simulink model "ModelD"  (R2014a)
settings: Solver=FixedStepDiscrete  StartTime=0.0  StopTime=10.0  RelTol=1e-3
libraries: simulink x8
settings Model: SimulationMode=external  ExtModeTrigDuration=100  Creator=admin  LastModifiedBy=admin
settings SolverCC: AutoInsertRateTranBlk=on
settings DataIOCC: SaveOutput=off  SaveTime=off
settings OptimizationCC: InlineParams=on  InlineInvariantSignals=on  StateBitsets=on  DataBitsets=on  UseTempVars=on  ZeroExternalMemoryAtStartup=off  ZeroInternalMemoryAtStartup=off  NoFixptDivByZeroProtection=on  EfficientFloat2IntCast=on  OptimizeModelRefInitCode=on  LifeSpan=1
settings DebuggingCC: SolverPrmCheckMsg=none
settings HardwareCC: ProdLargestAtomicInteger=Long  ProdLargestAtomicFloat=Double  ProdEndianess=LittleEndian  ProdHWDeviceType=ARM Compatible->ARM Cortex
settings RTWCC: SystemTargetFile=realtime.tlc  TLCOptions=-p0  GenCodeOnly=on  GenerateMakefile=off  TemplateMakefile=realtime.tmf  Description=Run on Target Hardware  RTWVerbose=off  ProcessScript=realtime_make_rtw_hook  IncludeHyperlinkInReport=on
settings CodeAppCC: ForceParamTrailComments=on  SimulinkDataObjDesc=on  CustomSymbolStrGlobalVar=rt$N$M  CustomSymbolStrType=$N$M  CustomSymbolStrFcn=$N$M$F  CustomSymbolStrMacro=$N$M  InsertBlockDesc=on
settings STFCustomTargetCC: TargetLibSuffix=.a  GenerateSampleERTMain=on  ConcurrentExecutionCompliant=off  GeneratePreprocessorConditionals=Use local settings  ERTCustomFileBanners=on  SupportNonInlinedSFcns=off  SupportVariableSizeSignals=on  MATLABClassNameForMDSCustomization=Simulink.SoftwareTarget.ERTCustomization  GRTInterface=off  SystemTargetFile=realtime.tlc
settings ERTTargetCC: CombineOutputUpdateFcns=off  SupportContinuousTime=on  SupportVariableSizeSignals=on  ExtModeMexArgs='localhost' 0 17725  ERTSrcFileBannerTemplate=realtime_code_template.cgt  ERTHdrFileBannerTemplate=realtime_code_template.cgt  ERTDataSrcFileTemplate=realtime_code_template.cgt  ERTDataHdrFileTemplate=realtime_code_template.cgt  ERTCustomFileTemplate=realtime_file_process.tlc

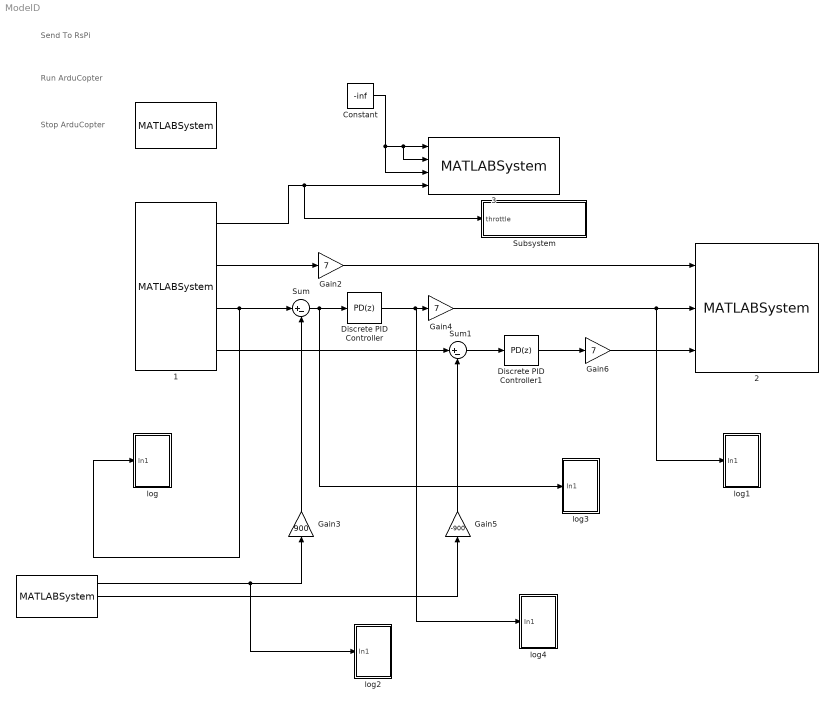
== system ModelD ==
  note: Send To RsPi
  note: Run ArduCopter
  note: Stop ArduCopter
  "  " : MATLABSystem  System=Gyro  SimulateUsing=Interpreted execution
      mask Type: Gyro
      mask Display:
      | disp('Gyro');
      | port_label('output',1,'x');
      | port_label('output',2,'y');
      | port_label('output',3,'z');
  "   " : MATLABSystem  System=Accel  SimulateUsing=Interpreted execution
      mask Type: Accel
      mask Display:
      | disp('Accel');
      | port_label('output',1,'x');
      | port_label('output',2,'y');
      | port_label('output',3,'z');
  "   1" : MATLABSystem  System=RC  SimulateUsing=Interpreted execution
      mask Type: RC
      mask Display:
      | disp('RC');
      | port_label('output',1,'thort');
      | port_label('output',2,'yawR');
      | port_label('output',3,'pitch');
      | port_label('output',4,'roll');
  "   2" : MATLABSystem  System=RateController  SimulateUsing=Interpreted execution
      mask Type: RateController
      mask Display:
      | disp('RateController');
      | port_label('input',1,'yaw');
      | port_label('input',2,'pitch');
      | port_label('input',3,'roll');
  "   3" : MATLABSystem  System=Motors  SimulateUsing=Interpreted execution
      mask Type: Motors
      mask Display:
      | disp('Motors');
      | port_label('input',1,'roll');
      | port_label('input',2,'pitch');
      | port_label('input',3,'yaw');
      | port_label('input',4,'throttle');
  Constant : Constant  Value=-inf
  Discrete PID Controller : simulink/Continuous/PID Controller  Controller=PD  TimeDomain=Discrete-time  SampleTime=-1  IntegratorMethod=Forward Euler  FilterMethod=Forward Euler  Form=Parallel  P=1  I=0  D=0.1  N=3  InitialConditionSource=internal  InitialConditionForIntegrator=0  InitialConditionForFilter=0  ExternalReset=none  ZeroCross=off  LimitOutput=off  UpperSaturationLimit=inf  LowerSaturationLimit=-inf  LinearizeAsGain=off  AntiWindupMode=none  Kb=1  TrackingMode=off  Kt=1  PParamMin=[]  PParamMax=[]  IParamMin=[]  IParamMax=[]  DParamMin=[]  DParamMax=[]  NParamMin=[]  NParamMax=[]  KbParamMin=[]  KbParamMax=[]  KtParamMin=[]  KtParamMax=[]  POutMin=[]  POutMax=[]  IOutMin=[]  IOutMax=[]  DOutMin=[]  DOutMax=[]  NOutMin=[]  NOutMax=[]  KbOutMin=[]  KbOutMax=[]  KtOutMin=[]  KtOutMax=[]  IntegratorOutMin=[]  IntegratorOutMax=[]  FilterOutMin=[]  FilterOutMax=[]  SumOutMin=[]  SumOutMax=[]  SumI1OutMin=[]  SumI1OutMax=[]  SumI2OutMin=[]  SumI2OutMax=[]  SumI3OutMin=[]  SumI3OutMax=[]  SumDOutMin=[]  SumDOutMax=[]  SaturationOutMin=[]  SaturationOutMax=[]  IntegratorContinuousStateAttributes=''  IntegratorStateMustResolveToSignalObject=off  IntegratorRTWStateStorageClass=Auto  FilterContinuousStateAttributes=''  FilterStateMustResolveToSignalObject=off  FilterRTWStateStorageClass=Auto
  Discrete PID Controller1 : simulink/Continuous/PID Controller  Controller=PD  TimeDomain=Discrete-time  SampleTime=-1  IntegratorMethod=Forward Euler  FilterMethod=Forward Euler  Form=Parallel  P=1  I=0  D=0.1  N=3  InitialConditionSource=internal  InitialConditionForIntegrator=0  InitialConditionForFilter=0  ExternalReset=none  ZeroCross=off  LimitOutput=off  UpperSaturationLimit=inf  LowerSaturationLimit=-inf  LinearizeAsGain=off  AntiWindupMode=none  Kb=1  TrackingMode=off  Kt=1  PParamMin=[]  PParamMax=[]  IParamMin=[]  IParamMax=[]  DParamMin=[]  DParamMax=[]  NParamMin=[]  NParamMax=[]  KbParamMin=[]  KbParamMax=[]  KtParamMin=[]  KtParamMax=[]  POutMin=[]  POutMax=[]  IOutMin=[]  IOutMax=[]  DOutMin=[]  DOutMax=[]  NOutMin=[]  NOutMax=[]  KbOutMin=[]  KbOutMax=[]  KtOutMin=[]  KtOutMax=[]  IntegratorOutMin=[]  IntegratorOutMax=[]  FilterOutMin=[]  FilterOutMax=[]  SumOutMin=[]  SumOutMax=[]  SumI1OutMin=[]  SumI1OutMax=[]  SumI2OutMin=[]  SumI2OutMax=[]  SumI3OutMin=[]  SumI3OutMax=[]  SumDOutMin=[]  SumDOutMax=[]  SaturationOutMin=[]  SaturationOutMax=[]  IntegratorContinuousStateAttributes=''  IntegratorStateMustResolveToSignalObject=off  IntegratorRTWStateStorageClass=Auto  FilterContinuousStateAttributes=''  FilterStateMustResolveToSignalObject=off  FilterRTWStateStorageClass=Auto
  Gain2 : Gain  Gain=7
  Gain3 : Gain  Gain=900
  Gain4 : Gain  Gain=7
  Gain5 : Gain  Gain=-900
  Gain6 : Gain  Gain=7
  Subsystem : Subsystem
      mask Display: fprintf('Check throttle range')
  Sum : Sum  Inputs=|+-
  Sum1 : Sum  Inputs=|+-
  log : Subsystem
  log1 : Subsystem
  log2 : Subsystem
  log3 : Subsystem
  log4 : Subsystem
  wires:
  "   1"/2 -> Gain2/1
  "   1"/3 -> log/1(In1), Sum/1
  Constant/1 -> "   3"/3, "   3"/2, "   3"/1
  "   1"/1 -> Subsystem/1(throttle), "   3"/4
  Gain2/1 -> "   2"/1
  "   "/1 -> log2/1(In1), Gain3/1
  Gain3/1 -> Sum/2
  Sum/1 -> log3/1(In1), Discrete PID Controller/1
  Discrete PID Controller/1 -> log4/1(In1), Gain4/1
  Gain4/1 -> log1/1(In1), "   2"/2
  "   1"/4 -> Sum1/1
  "   "/2 -> Gain5/1
  Gain5/1 -> Sum1/2
  Sum1/1 -> Discrete PID Controller1/1
  Discrete PID Controller1/1 -> Gain6/1
  Gain6/1 -> "   2"/3

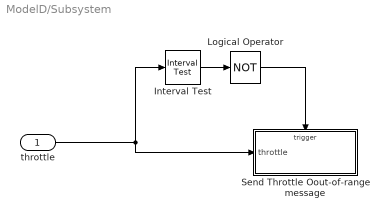
== system ModelD/Subsystem ==
  throttle : Inport
  Interval Test : simulink/Logic and Bit Operations/Interval Test  IntervalClosedRight=on  uplimit=0  IntervalClosedLeft=on  lowlimit=1000  OutDataTypeStr=boolean
  Logical Operator : Logic  Operator=NOT  AllPortsSameDT=off  OutDataTypeStr=boolean
  Send Throttle Oout-of-range message : Subsystem  TreatAsAtomicUnit=on
  wires:
  throttle/1 -> Interval Test/1, Send Throttle Oout-of-range message/1(throttle)
  Logical Operator/1 -> Send Throttle Oout-of-range message/Trigger
  Interval Test/1 -> Logical Operator/1

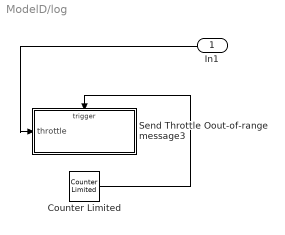
== system ModelD/log ==
  In1 : Inport
  Counter Limited : simulink/Sources/Counter Limited  uplimit=400  tsamp=-1
  Send Throttle Oout-of-range message3 : Subsystem  TreatAsAtomicUnit=on
  wires:
  Counter Limited/1 -> Send Throttle Oout-of-range message3/Trigger
  In1/1 -> Send Throttle Oout-of-range message3/1(throttle)

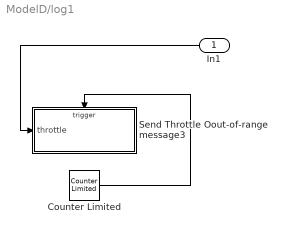
== system ModelD/log1 ==
  In1 : Inport
  Counter Limited : simulink/Sources/Counter Limited  uplimit=400  tsamp=-1
  Send Throttle Oout-of-range message3 : Subsystem  TreatAsAtomicUnit=on
  wires:
  In1/1 -> Send Throttle Oout-of-range message3/1(throttle)
  Counter Limited/1 -> Send Throttle Oout-of-range message3/Trigger

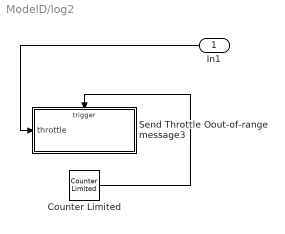
== system ModelD/log2 ==
  In1 : Inport
  Counter Limited : simulink/Sources/Counter Limited  uplimit=400  tsamp=-1
  Send Throttle Oout-of-range message3 : Subsystem  TreatAsAtomicUnit=on
  wires:
  Counter Limited/1 -> Send Throttle Oout-of-range message3/Trigger
  In1/1 -> Send Throttle Oout-of-range message3/1(throttle)

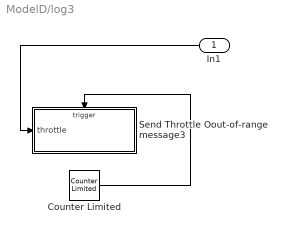
== system ModelD/log3 ==
  In1 : Inport
  Counter Limited : simulink/Sources/Counter Limited  uplimit=400  tsamp=-1
  Send Throttle Oout-of-range message3 : Subsystem  TreatAsAtomicUnit=on
  wires:
  In1/1 -> Send Throttle Oout-of-range message3/1(throttle)
  Counter Limited/1 -> Send Throttle Oout-of-range message3/Trigger

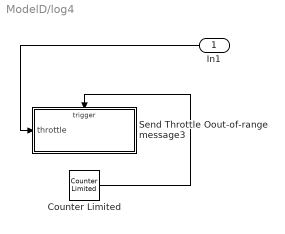
== system ModelD/log4 ==
  In1 : Inport
  Counter Limited : simulink/Sources/Counter Limited  uplimit=400  tsamp=-1
  Send Throttle Oout-of-range message3 : Subsystem  TreatAsAtomicUnit=on
  wires:
  Counter Limited/1 -> Send Throttle Oout-of-range message3/Trigger
  In1/1 -> Send Throttle Oout-of-range message3/1(throttle)

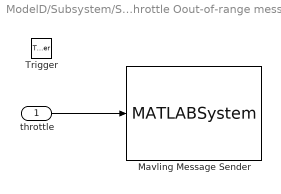
== system ModelD/Subsystem/Send Throttle Oout-of-range message ==
  throttle : Inport
  Trigger : TriggerPort
  Mavling Message Sender : MATLABSystem  System=MavlinkMsg  Message=throttle not between 0 to 1:
      mask Type: MavlinkMsg
      mask Display:
      | disp('MavlinkMsg');
      | port_label('input',1,'u');
  wires:
  throttle/1 -> Mavling Message Sender/1

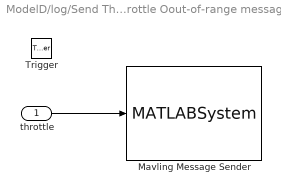
== system ModelD/log/Send Throttle Oout-of-range message3 ==
  throttle : Inport
  Trigger : TriggerPort
  Mavling Message Sender : MATLABSystem  System=MavlinkMsg  Message=rc pitch:
      mask Type: MavlinkMsg
      mask Display:
      | disp('MavlinkMsg');
      | port_label('input',1,'u');
  wires:
  throttle/1 -> Mavling Message Sender/1

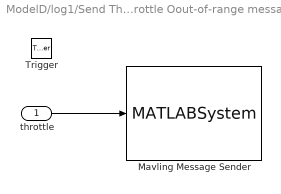
== system ModelD/log1/Send Throttle Oout-of-range message3 ==
  throttle : Inport
  Trigger : TriggerPort
  Mavling Message Sender : MATLABSystem  System=MavlinkMsg  Message=rate cont. pitch:
      mask Type: MavlinkMsg
      mask Display:
      | disp('MavlinkMsg');
      | port_label('input',1,'u');
  wires:
  throttle/1 -> Mavling Message Sender/1

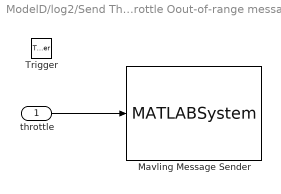
== system ModelD/log2/Send Throttle Oout-of-range message3 ==
  throttle : Inport
  Trigger : TriggerPort
  Mavling Message Sender : MATLABSystem  System=MavlinkMsg  Message=Accel. x:
      mask Type: MavlinkMsg
      mask Display:
      | disp('MavlinkMsg');
      | port_label('input',1,'u');
  wires:
  throttle/1 -> Mavling Message Sender/1

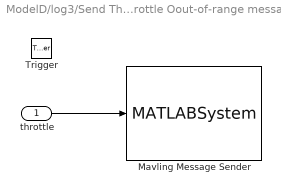
== system ModelD/log3/Send Throttle Oout-of-range message3 ==
  throttle : Inport
  Trigger : TriggerPort
  Mavling Message Sender : MATLABSystem  System=MavlinkMsg  Message=befor PID:
      mask Type: MavlinkMsg
      mask Display:
      | disp('MavlinkMsg');
      | port_label('input',1,'u');
  wires:
  throttle/1 -> Mavling Message Sender/1

== system ModelD/log4/Send Throttle Oout-of-range message3 ==
  throttle : Inport
  Trigger : TriggerPort
  Mavling Message Sender : MATLABSystem  System=MavlinkMsg  Message=After PID:
      mask Type: MavlinkMsg
      mask Display:
      | disp('MavlinkMsg');
      | port_label('input',1,'u');
  wires:
  throttle/1 -> Mavling Message Sender/1
